simulink model "test"  (R2021a)
settings: Solver=FixedStepAuto  StartTime=0.0  StopTime=inf  RelTol=1e-3
PreLoadFcn:
  | run("~/youbot_state_machine/subtasks.m")
model workspace: external: MAT-File /home/zxc/youbot_state_machine/subtuskseq.mat (data not in the file)
undefined symbols (not defined in the file or in its folder): Goal, GoalId, Header, Pose
libraries: robotlib x6
settings Model: OrderedModelArguments=off  Creator=zxc  LastModifiedBy=zxc
settings OptimizationCC: EnhancedBackFolding=on  PassReuseOutputArgsAs=Individual arguments  ZeroExternalMemoryAtStartup=off  ZeroInternalMemoryAtStartup=off  MaxStackSize=64  OptimizeBlockOrder=speed  DifferentSizesBufferReuse=on  OptimizationCustomize=off  EfficientTunableParamExpr=on
settings DebuggingCC: ParameterTunabilityLossMsg=error
settings HardwareCC: ProdBitPerPointer=32  ProdBitPerSizeT=32  ProdBitPerPtrDiffT=32  ProdLargestAtomicFloat=None  ProdIntDivRoundTo=Undefined  ProdEndianess=Unspecified  ProdWordSize=32  ProdHWDeviceType=Generic->Unspecified (assume 32-bit Generic)  UseEmbeddedCoderFeatures=off
settings SFSimCC: MATLABDynamicMemAlloc=off
settings RTWCC: SystemTargetFile=ert.tlc  HardwareBoard=Robot Operating System (ROS)  TLCOptions="-aInlineSetEventsForThisBaseRateFcn=TLC_FALSE -aSuppressMultiTaskScheduler=TLC_FALSE  -aRateBasedStepFcn=0"  TemplateMakefile=ert_default_tmf  Toolchain=Catkin  TargetLang=C++
settings CodeAppCC: ForceParamTrailComments=on  IgnoreCustomStorageClasses=off  OperatorAnnotations=on  SimulinkDataObjDesc=on  SFDataObjDesc=on  InsertBlockDesc=on
settings ERTTargetCC: SupportNonInlinedSFcns=on

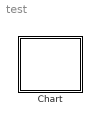
== system test ==
  Chart : Stateflow chart  TreatAsAtomicUnit=on

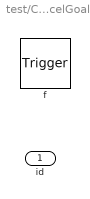
== system test/Chart/cancelGoal ==
  id : Inport  OutDataTypeStr=double  PortDimensions=1
  f : TriggerPort  TriggerType=function-call  VariantControl=(inherit)
      settings: CopyFcn=Stateflow.SLINSF.SimulinkMan.removeBlockPreDeleteFcn  PreDeleteFcn=Stateflow.SLINSF.SimulinkMan.unsafePredeleteFcn

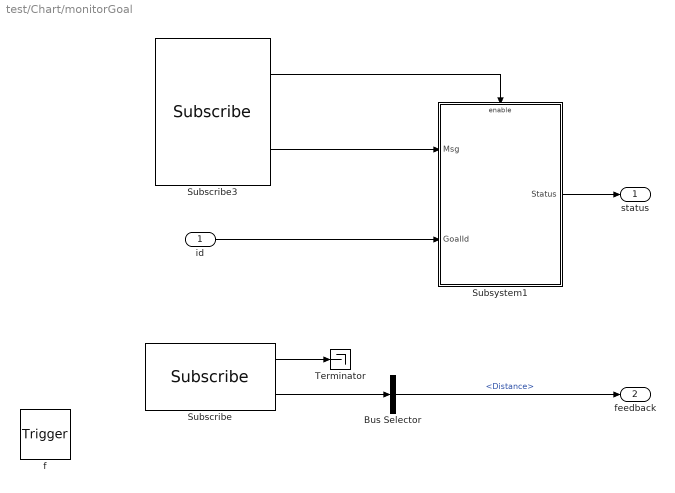
== system test/Chart/monitorGoal ==
  id : Inport  OutDataTypeStr=Bus: SubtaskSequence  PortDimensions=1
  f : TriggerPort  TriggerType=function-call  VariantControl=(inherit)
      settings: CopyFcn=Stateflow.SLINSF.SimulinkMan.removeBlockPreDeleteFcn  PreDeleteFcn=Stateflow.SLINSF.SimulinkMan.unsafePredeleteFcn
  Bus Selector : BusSelector  OutputSignals=Feedback.Distance
  Subscribe : robotlib/Subscribe  topicSource=Select from ROS network  topic=/motion_controller_node/feedback  messageType=motion_controller/motion_controllerActionFeedback  SampleTime=-1  legacyBusStruct=off  messageQueueLength=1
      settings: SourceProductBaseCode=RO
  Subscribe3 : robotlib/Subscribe  topicSource=Select from ROS network  topic=/motion_controller_node/status  messageType=actionlib_msgs/GoalStatusArray  SampleTime=-1  legacyBusStruct=off  messageQueueLength=1
  Subsystem1 : Subsystem
  Terminator : Terminator
  status : Outport
  feedback : Outport  Port=2
  wires:
  Bus Selector/1 -> feedback/1  "<Distance>"
  Subsystem1/1(Status) -> status/1
  Subscribe/1 -> Terminator/1
  Subscribe3/2 -> Subsystem1/1(Msg)
  Subscribe/2 -> Bus Selector/1
  Subscribe3/1 -> Subsystem1/Enable
  id/1 -> Subsystem1/2(GoalId)

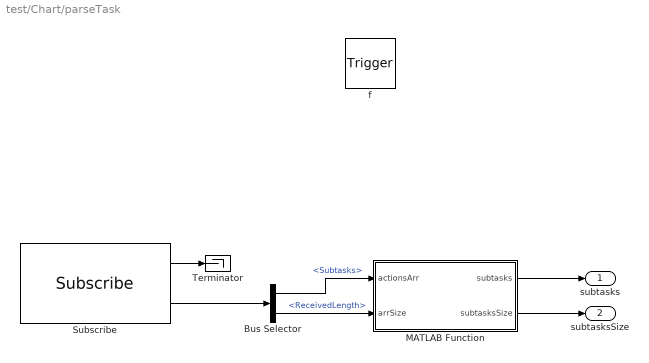
== system test/Chart/parseTask ==
  f : TriggerPort  TriggerType=function-call  VariantControl=(inherit)
      settings: CopyFcn=Stateflow.SLINSF.SimulinkMan.removeBlockPreDeleteFcn  PreDeleteFcn=Stateflow.SLINSF.SimulinkMan.unsafePredeleteFcn
  Bus Selector : BusSelector  OutputSignals=Subtasks,Subtasks_SL_Info.ReceivedLength
  MATLAB Function : MATLAB Function  TreatAsAtomicUnit=on
  Subscribe : robotlib/Subscribe  topicSource=Select from ROS network  topic=/atwork_commander/object_task  messageType=atwork_commander_msgs/ObjectTask  SampleTime=-1  legacyBusStruct=off  messageQueueLength=1
  Terminator : Terminator
  subtasks : Outport
  subtasksSize : Outport  Port=2
  wires:
  Subscribe/2 -> Bus Selector/1
  Bus Selector/1 -> MATLAB Function/1(actionsArr)  "<Subtasks>"
  Bus Selector/2 -> MATLAB Function/2(arrSize)  "<ReceivedLength>"
  MATLAB Function/2(subtasksSize) -> subtasksSize/1
  MATLAB Function/1(subtasks) -> subtasks/1
  Subscribe/1 -> Terminator/1

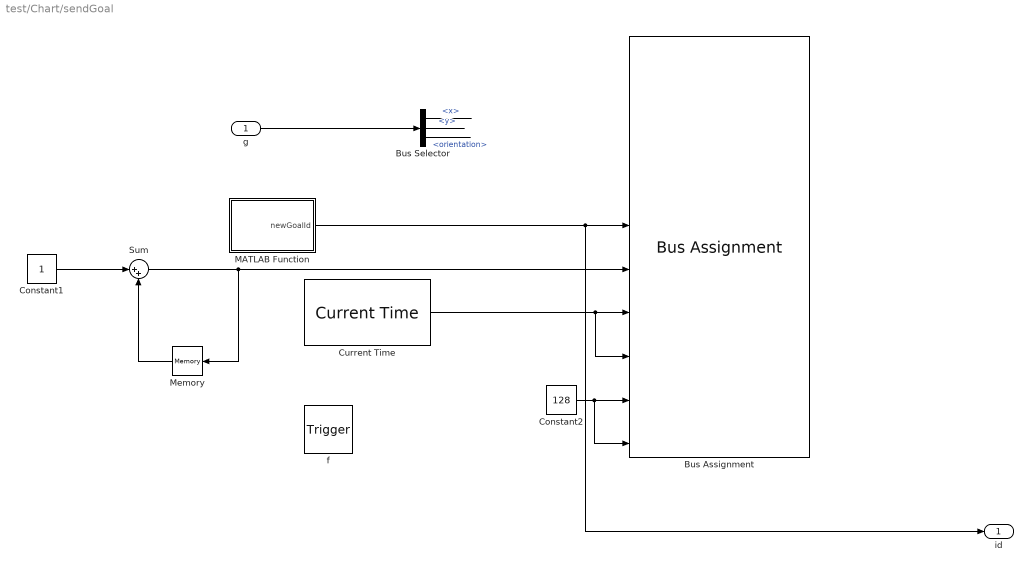
== system test/Chart/sendGoal ==
  g : Inport  OutDataTypeStr=Bus: SubtaskSequence  PortDimensions=1
  f : TriggerPort  TriggerType=function-call  VariantControl=(inherit)
      settings: CopyFcn=Stateflow.SLINSF.SimulinkMan.removeBlockPreDeleteFcn  PreDeleteFcn=Stateflow.SLINSF.SimulinkMan.unsafePredeleteFcn
  Bus Assignment : BusAssignment  AssignedSignals=Goal.NextPos.Linear.X,Goal.NextPos.Linear.Y,Goal.NextPos.Angular.Z,GoalId.Id,Header.Seq,Header.Stamp,GoalId.Stamp,GoalId.Id_SL_Info.CurrentLength,GoalId.Id_SL_Info.ReceivedLength
  Bus Selector : BusSelector  OutputSignals=x,y,orientation
  Constant1 : Constant  OutDataTypeStr=uint32
  Constant2 : Constant  Value=128  OutDataTypeStr=uint32
  Current Time : robotlib/Current Time  OutputFormat=bus  SampleTime=-1  ModelName=SimulinkActionClientStateFlow
      settings: SourceProductBaseCode=RO
  MATLAB Function : MATLAB Function  TreatAsAtomicUnit=on
  Memory : Memory  InitialCondition=1  InheritSampleTime=on
  Sum : Sum  Inputs=|++
  id : Outport
  wires:
  Memory/1 -> Sum/2
  Current Time/1 -> Bus Assignment/7, Bus Assignment/8
  Constant1/1 -> Sum/1
  Sum/1 -> Bus Assignment/6, Memory/1
  Constant2/1 -> Bus Assignment/10, Bus Assignment/9
  MATLAB Function/1(newGoalId) -> id/1, Bus Assignment/5
  g/1 -> Bus Selector/1
  Bus Selector/2 -> ?  "<y>"
  Bus Selector/1 -> ?  "<x>"
  Bus Selector/3 -> ?  "<orientation>"

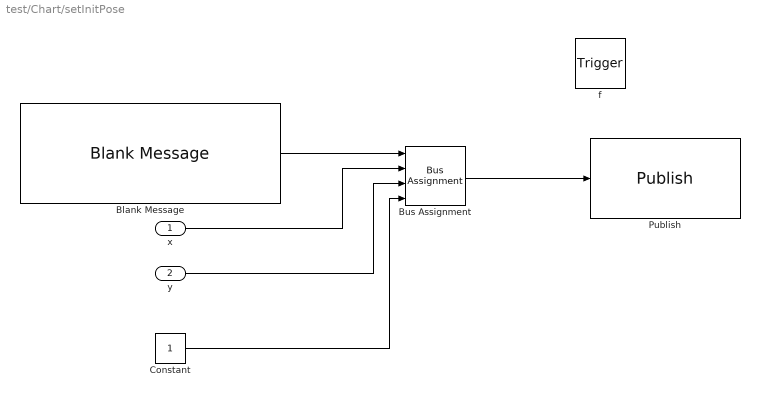
== system test/Chart/setInitPose ==
  x : Inport  OutDataTypeStr=double  PortDimensions=1
  y : Inport  Port=2  OutDataTypeStr=double  PortDimensions=1
  f : TriggerPort  TriggerType=function-call  VariantControl=(inherit)
      settings: CopyFcn=Stateflow.SLINSF.SimulinkMan.removeBlockPreDeleteFcn  PreDeleteFcn=Stateflow.SLINSF.SimulinkMan.unsafePredeleteFcn
  Blank Message : robotlib/Blank Message  messageClass=Message  entityType=geometry_msgs/PoseWithCovarianceStamped  messageType=geometry_msgs/PoseWithCovarianceStamped  SampleTime=inf  legacyBusStruct=off
  Bus Assignment : BusAssignment  AssignedSignals=Pose.Pose.Position.X,Pose.Pose.Position.Y,Pose.Pose.Orientation.W
  Constant : Constant
  Publish : robotlib/Publish  topicSource=Specify your own  topic=/initialpose  messageType=geometry_msgs/PoseWithCovarianceStamped  legacyBusStruct=off  messageQueueLength=1
  wires:
  Blank Message/1 -> Bus Assignment/1
  Bus Assignment/1 -> Publish/1
  x/1 -> Bus Assignment/2
  y/1 -> Bus Assignment/3
  Constant/1 -> Bus Assignment/4

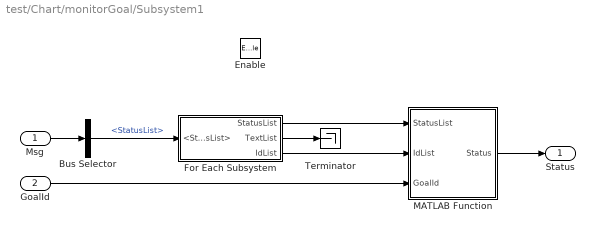
== system test/Chart/monitorGoal/Subsystem1 ==
  Msg : Inport
  GoalId : Inport  Port=2
  Enable : EnablePort
  Bus Selector : BusSelector  OutputSignals=StatusList
  For Each Subsystem : Subsystem  TreatAsAtomicUnit=on
  MATLAB Function : MATLAB Function  TreatAsAtomicUnit=on
  Terminator : Terminator
  Status : Outport  VectorParamsAs1DForOutWhenUnconnected=off
  wires:
  Bus Selector/1 -> For Each Subsystem/1(<StatusList>)  "<StatusList>"
  Msg/1 -> Bus Selector/1
  For Each Subsystem/1(StatusList) -> MATLAB Function/1(StatusList)
  For Each Subsystem/3(IdList) -> MATLAB Function/2(IdList)
  GoalId/1 -> MATLAB Function/3(GoalId)
  MATLAB Function/1(Status) -> Status/1
  For Each Subsystem/2(TextList) -> Terminator/1

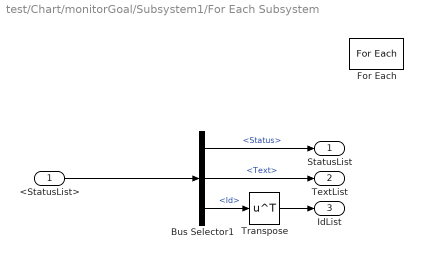
== system test/Chart/monitorGoal/Subsystem1/For Each Subsystem ==
  <StatusList> : Inport  Partition=on  PartitionDimension=1  PartitionWidth=1  PartitionOffset=0
  Bus Selector1 : BusSelector  OutputSignals=Status,Text,GoalId.Id
  For Each : ForEach  DisableCoverage=on
  Transpose : Math  Operator=transpose  SignedPower=on  SaturateOnIntegerOverflow=on
  StatusList : Outport  ConcatenationDimension=1
  TextList : Outport  Port=2  ConcatenationDimension=1
  IdList : Outport  Port=3  ConcatenationDimension=1
  wires:
  Bus Selector1/2 -> TextList/1  "<Text>"
  Bus Selector1/1 -> StatusList/1  "<Status>"
  <StatusList>/1 -> Bus Selector1/1
  Bus Selector1/3 -> Transpose/1  "<Id>"
  Transpose/1 -> IdList/1

== matlab function test/Chart/parseTask/MATLAB Function ==
  data: subtasks output Bus: SubtaskSequence; actionsArr input; arrSize input; subtasksSize output
function [subtasks, subtasksSize] = fcn(actionsArr, arrSize)
 
  function goToPlace = moveToSourcePlaceSubtask(action, placesArr)
       goToPlace.subtaskCode = 1;
       goToPlace.x = 0;
       goToPlace.y = 0;
       goToPlace.orientation = 0;
       goToPlace.objectCode = 0;
       goToPlace.objectCavity = 0;
               
       
       placeName = blanks(4);
       for ch = 1:action.Source_SL_Info.ReceivedLength 
            placeName(ch) = char(action.Source(ch));
       end
       
       for place = 1:length(placesArr)
           if strcmp(placeName, placesArr(place).name)
               goToPlace.x = placesArr(place).x;
               goToPlace.y = placesArr(place).y;
               goToPlace.orientation = placesArr(place).orientation;         
           end
       end
  end
  
  function goToPlace = moveToDestinationPlaceSubtask(action, placesArr)
       goToPlace.subtaskCode = 1;
       goToPlace.x = 0;
       goToPlace.y = 0;
       goToPlace.orientation = 0;
       goToPlace.objectCode = 0;
       goToPlace.objectCavity = 0;
               
       
       placeName = blanks(4);
       for ch = 1:action.Destination_SL_Info.ReceivedLength 
            placeName(ch) = char(action.Destination(ch));
       end
       
       for place = 1:length(placesArr)
           if strcmp(placeName, placesArr(place).name)
               goToPlace.x = placesArr(place).x;
               goToPlace.y = placesArr(place).y;
               goToPlace.orientation = placesArr(place).orientation;         
           end
       end
  end

  function goGrasp = graspSubtask(obj)
       goGrasp.subtaskCode = 2;
       goGrasp.x = 0;
       goGrasp.y = 0;
       goGrasp.orientation = 0;
       goGrasp.objectCode = double(obj);
       goGrasp.objectCavity = 0;
  end

  function goDeliver = deliverSubtask(obj, objState)
       goDeliver.subtaskCode = 3;
       goDeliver.x = 0;
       goDeliver.y = 0;
       goDeliver.orientation = 0;
       goDeliver.objectCode = double(obj);
       goDeliver.objectCavity = double(objState);
  end
    
WS01.name = 'WS01';
WS01.x = 0.1;
WS01.y = 0.2;
WS01.orientation = 45;

WS02.name = 'WS02';
WS02.x = 0.1;
WS02.y = 0.2;
WS02.orientation = 45;

PP01.name = 'PP01';
PP01.x = 0.1;
PP01.y = 0.2;
PP01.orientation = 45;

placesPositions = [WS01 WS02 PP01];

subtuskTemplate.subtaskCode = 0;
subtuskTemplate.x = 0;
subtuskTemplate.y = 0;
subtuskTemplate.orientation = 0;
subtuskTemplate.objectCode = 0;
subtuskTemplate.objectCavity = 0;
subtasksSize = 0;

structArr = repmat(subtuskTemplate,100,1);

currIdx = 1;
       
for i = 1:arrSize 
   m1 = moveToSourcePlaceSubtask(actionsArr(i), placesPositions);
   structArr(currIdx) = m1;
   currIdx = currIdx + 1;
   
   g1 = graspSubtask(actionsArr(i).Object.Object_);
   structArr(currIdx) = g1;
   currIdx = currIdx + 1;
       
   m2 = moveToDestinationPlaceSubtask(actionsArr(i), placesPositions);
   structArr(currIdx) = m2;
   currIdx = currIdx + 1;
       
   d1 = deliverSubtask(actionsArr(i).Object.Object_, actionsArr(i).Object.Target);
   structArr(currIdx) = d1;
   currIdx = currIdx + 1;
       
end

subtasksSize = currIdx - 1;
subtasks = structArr;
end

== matlab function test/Chart/sendGoal/MATLAB Function ==
  data: newGoalId output
function newGoalId = genRandGoalId()

newGoalId = uint8(rand(1,128)*25)+65;

== stateflow chart test/Chart ==
  state setInitPose(x,y) [function]
  state Init
    en: setInitPose(0.5, 1);
  state [status,feedback] = monitorGoal(id) [function]
  state id = sendGoal(g) [function]
  state cancelGoal(id) [function] [commented out]
  state WaitSubtasks
    en: step = 1
    en: subtasksSize = 0
    du: [subtasks,  subtasksSize] = parseTask();
  state NextSubtask
    en: nextSubtask = subtasks(step)
    en: step = step +1
  state Move
    en: goalID = sendGoal(nextSubtask);
    en, du: [MoveStatus, MoveFeedback] = monitorGoal(goalID);
    en, du: disp(MoveFeedback)
  state Grasp
    en: goalID = sendGoal(nextSubtask);
    en, du: [GraspStatus, GraspFeedback] = monitorGoal(goalID);
    en, du: disp(GraspFeedback)
  state [subtasks, subtasksSize] = parseTask [function]
  state Deliver
    en: goalID = sendGoal(nextSubtask);
    en, du: [DeliverStatus, DeliverFeedback] = monitorGoal(goalID);
    en, du: disp(DeliverFeedback)
  state Finished
    en: disp("FINISHED")
  state Error
    en: disp("ERROR")
  (default) -> Init
  Init -> WaitSubtasks
  NextSubtask -> Move [order 3] : [nextSubtask.subtaskCode == 1]
  Move -> Error [order 2] : [MoveStatus == 2 || MoveStatus == 4 || MoveStatus == 5]
  Move -> NextSubtask [order 1] : [MoveStatus == 3]
  WaitSubtasks -> NextSubtask : [subtasksSize ~= 0]
  Grasp -> Error [order 2] : [GraspStatus == 2 || GraspStatus == 4 || GraspStatus == 5]
  NextSubtask -> Grasp [order 2] : [nextSubtask.subtaskCode == 2]
  Grasp -> NextSubtask [order 1] : [GraspStatus == 3]
  Deliver -> Error [order 2] : [DeliverStatus == 2 || DeliverStatus == 4 || DeliverStatus == 5]
  NextSubtask -> Deliver [order 4] : [nextSubtask.subtaskCode == 3]
  Deliver -> NextSubtask [order 1] : [DeliverStatus == 3]
  NextSubtask -> Finished [order 1] : [nextSubtask.subtaskCode == 0]
  data: x function_input double size=1; y function_input double size=1; id function_input Bus: SubtaskSequence size=1; status function_output; feedback function_output; g function_input Bus: SubtaskSequence size=1; id function_output; id function_input double size=1; subtasks function_output; subtasksSize function_output; subtasks local Bus: SubtaskSequence size=100; step local int32; subtasksSize local double; answer local double; nextSubtask local Bus: SubtaskSequence

== matlab function test/Chart/monitorGoal/Subsystem1/MATLAB Function ==
  data: StatusList input; Status output; IdList input; GoalId input
function Status  = fcn(StatusList, IdList, GoalId)
Status = uint8(0);
for ii = 1:16 % Size of IdList - could also be managed
    if GoalId == IdList(ii,:)
        Status = StatusList(ii,:);
        break;
    end
end
